simulink model "Disturbance_Stabilization_Simulink_Offline_Pendulum_Control"  (R2022b)
settings: Solver=VariableStepAuto  StartTime=0.0  StopTime=30  RelTol=1e-3
undefined symbols (not defined in the file): A, A_ob, B, B_ob, C_full, C_ob, D_full, D_ob, Kpp, sigbuilder_block, voltage_max, x0
settings Model: Creator=utente  LastModifiedBy=federicocorso
settings SolverCC: AlgebraicLoopSolver=TrustRegion
settings DebuggingCC: UnconnectedInputMsg=warning  UnconnectedOutputMsg=warning  UnconnectedLineMsg=warning  SFMachineParentedDataDiag=warning
settings ModelReferenceCC: EnableRefExpFcnMdlSchedulingChecks=on

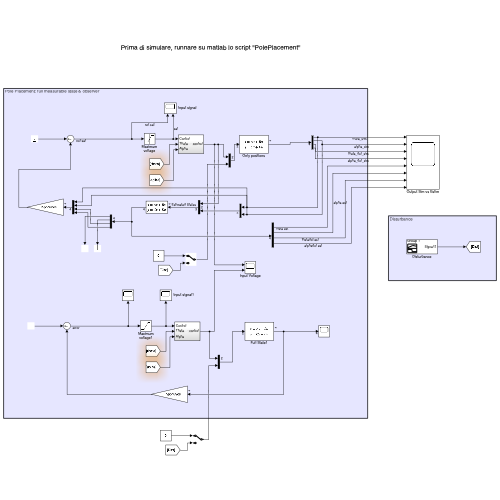
[thumbnail: Simulink's stored preview of the top-level diagram]
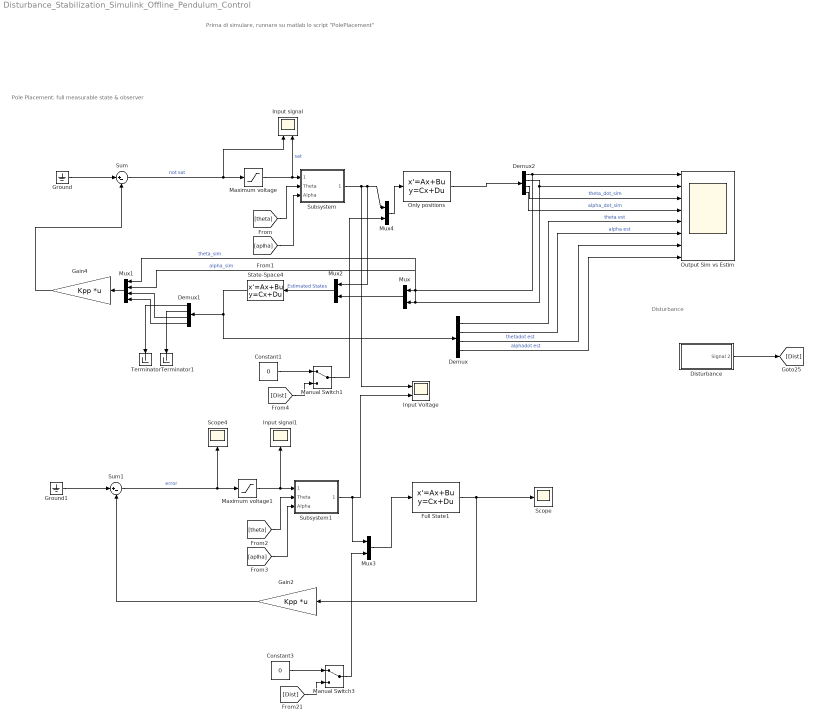
== system Disturbance_Stabilization_Simulink_Offline_Pendulum_Control ==
  note: Disturbance
  note: Pole Placement: full measurable state & observer
  note: Prima di simulare, runnare su matlab lo script "PolePlacement"
  Constant1 : Constant  Value=0
  Constant3 : Constant  Value=0
  Demux : Demux
  Demux1 : Demux
  Demux2 : Demux
  Disturbance : Subsystem  Tag=STV Subsys  LoadFcn=sigbuilder_block('load');  StartFcn=sigbuilder_block('start');  StopFcn=sigbuilder_block('stop');  ClipboardFcn=sigbuilder_block('clipboard');  mask(Sigbuilder block){tuvar=[0:10]}
      mask help: Simulink:masks:SigbuilderBlock_MD
      mask init:
      | if ~strcmp(get_param(bdroot(gcbh),'SimulationStatus'),'stopped') tuvar = sigbuilder_block('maskInit'); end
      settings: CopyFcn=sigbuilder_block('copy');  DeleteFcn=sigbuilder_block('delete');  ModelCloseFcn=sigbuilder_block('modelClose');  PreSaveFcn=sigbuilder_block('preSave');  PauseFcn=sigbuilder_block('pause');  ContinueFcn=sigbuilder_block('continue');  NameChangeFcn=sigbuilder_block('namechange');  OpenFcn=sigbuilder_block('open',[516 294 550 400 ]);  CloseFcn=sigbuilder_block('close');
      mask Display: plot(0, 0, 100, 100,[2, 2, 32, 32, 2], [68, 8, 8, 68, 68],[32, 2], [38, 38], [32, 19, 2],[53, 60, 44], [32, 17, 17, 2],[16, 16, 31, 31]);txt = getActiveGroup(gcbh);text(2, 100, txt,'verticalAlignment', 'top');
  Full State1 : StateSpace  A=A  B=B  C=C_full  D=D_full  InitialCondition=x0
  Gain2 : Gain  Gain=Kpp  Multiplication=Matrix(K*u) (u vector)
  Gain4 : Gain  Gain=Kpp  Multiplication=Matrix(K*u) (u vector)
  Ground : Ground
  Ground1 : Ground
  Input Voltage : Scope  NumInputPorts=2
  Input signal : Scope  NumInputPorts=2
  Input signal1 : Scope
  Manual Switch1 : ManualSwitch
  Manual Switch3 : ManualSwitch
  Maximum voltage : Saturate  UpperLimit=voltage_max  LowerLimit=-voltage_max
  Maximum voltage1 : Saturate  UpperLimit=voltage_max  LowerLimit=-voltage_max
  Mux{,2..4} (4 alike) : Mux  Inputs=2
  Mux1 : Mux
  Only positions : StateSpace  A=A  B=B  C=C_full  D=D_full  InitialCondition=x0
  Output Sim vs Estim : Scope  NumInputPorts=8
  Scope : Scope
  Scope4 : Scope
  State-Space4 : StateSpace  A=A_ob  B=B_ob  C=C_ob  D=D_ob  InitialCondition=[0;0;0;0]
  Subsystem : Subsystem
  Subsystem1 : Subsystem
  Sum : Sum  Inputs=|+-
  Sum1 : Sum  Inputs=|+-
  Terminator : Terminator
  Terminator1 : Terminator
  wires:
  Maximum voltage/1 -> Input signal/2, Subsystem/1(Control)  "sat"
  [theta] -> Subsystem/2(Theta)
  [aplha] -> Subsystem/3(Alpha)
  Ground/1 -> Sum/1
  Sum/1 -> Input signal/1, Maximum voltage/1  "not sat"
  Gain4/1 -> Sum/2
  Mux2/1 -> State-Space4/1  "Estimated States"
  State-Space4/1 -> Demux1/1, Demux/1
  Subsystem/1(control) -> Mux2/1, Mux4/1, Input Voltage/1
  Sum1/1 -> Maximum voltage1/1, Scope4/1  "error"
  Ground1/1 -> Sum1/1
  Full State1/1 -> Scope/1, Gain2/1
  Subsystem1/1(control) -> Input Voltage/2, Mux3/1
  Maximum voltage1/1 -> Input signal1/1, Subsystem1/1(Control)
  [aplha] -> Subsystem1/3(Alpha)
  [theta] -> Subsystem1/2(Theta)
  Gain2/1 -> Sum1/2
  Demux/1 -> Output Sim vs Estim/5  "theta est"
  Demux/2 -> Output Sim vs Estim/6  "alpha est"
  Demux/3 -> Output Sim vs Estim/7  "thetadot est"
  Demux/4 -> Output Sim vs Estim/8  "alphadot est"
  Only positions/1 -> Demux2/1
  Mux/1 -> Mux2/2
  Demux2/2 -> Output Sim vs Estim/2, Mux1/2, Mux/2  "alpha_sim"
  Demux2/1 -> Output Sim vs Estim/1, Mux1/1, Mux/1  "theta_sim"
  Demux2/3 -> Output Sim vs Estim/3  "theta_dot_sim"
  Demux2/4 -> Output Sim vs Estim/4  "alpha_dot_sim"
  Mux1/1 -> Gain4/1
  Demux1/3 -> Mux1/3
  Demux1/4 -> Mux1/4
  Demux1/1 -> Terminator/1
  Demux1/2 -> Terminator1/1
  Disturbance/1(Signal 2) -> [Dist]
  [Dist] -> Manual Switch3/2
  Manual Switch3/1 -> Mux3/2
  Constant3/1 -> Manual Switch3/1
  Mux3/1 -> Full State1/1
  Constant1/1 -> Manual Switch1/1
  [Dist] -> Manual Switch1/2
  Mux4/1 -> Only positions/1
  Manual Switch1/1 -> Mux4/2

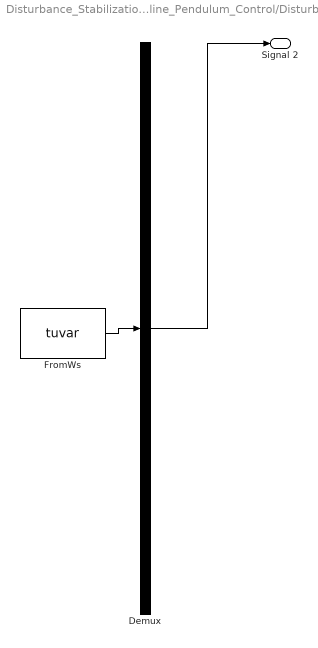
== system Disturbance_Stabilization_Simulink_Offline_Pendulum_Control/Disturbance ==
  Demux : Demux  Tag=STV Demux  Outputs=1
      settings: DisplayOption=none
  FromWs : FromWorkspace  Tag=STV FromWs  VariableName=tuvar
      SigBuilderData=|
      | common.afterFinalStr = 'Extrapolate'
      | common.sampleTime = 0
      | dataSet.timeRange = [0 10]
      | dataSet.name = 'Group 1'
      | sbobj.Groups.Name = 'Group 1'
      | sbobj.Groups.Signals.Name = 'Signal 2'
      | sbobj.Groups.Signals.XData = [0 4 4 4.01 4.01 10]
      | sbobj.Groups.Signals.YData = [0 0 0.2 0.2 0 0]
  Signal 2 : Outport  Tag=STV Outport
  wires:
  Demux/1 -> Signal 2/1
  FromWs/1 -> Demux/1

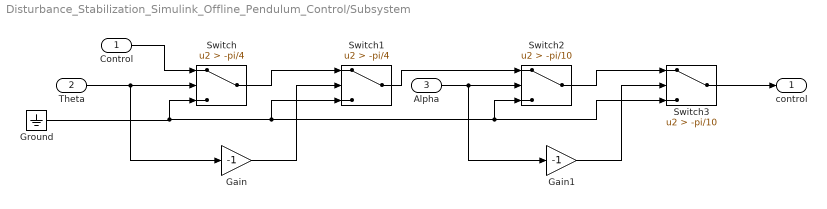
== system Disturbance_Stabilization_Simulink_Offline_Pendulum_Control/Subsystem ==
  Control : Inport
  Theta : Inport  Port=2
  Alpha : Inport  Port=3
  Gain : Gain  Gain=-1
  Gain1 : Gain  Gain=-1
  Ground : Ground
  Switch : Switch  Criteria=u2 > Threshold  Threshold=-pi/4  SaturateOnIntegerOverflow=off  InputSameDT=off
  Switch1 : Switch  Criteria=u2 > Threshold  Threshold=-pi/4  SaturateOnIntegerOverflow=off  InputSameDT=off
  Switch2 : Switch  Criteria=u2 > Threshold  Threshold=-pi/10  SaturateOnIntegerOverflow=off  InputSameDT=off
  Switch3 : Switch  Criteria=u2 > Threshold  Threshold=-pi/10  SaturateOnIntegerOverflow=off  InputSameDT=off
  control : Outport
  wires:
  Gain/1 -> Switch1/2
  Theta/1 -> Gain/1, Switch/2
  Control/1 -> Switch/1
  Switch/1 -> Switch1/1
  Gain1/1 -> Switch3/2
  Switch1/1 -> Switch2/1
  Ground/1 -> Switch3/3, Switch2/3, Switch1/3, Switch/3
  Switch2/1 -> Switch3/1
  Alpha/1 -> Switch2/2, Gain1/1
  Switch3/1 -> control/1

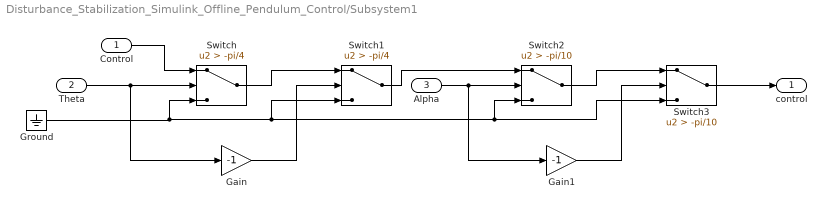
== system Disturbance_Stabilization_Simulink_Offline_Pendulum_Control/Subsystem1 ==
  Control : Inport
  Theta : Inport  Port=2
  Alpha : Inport  Port=3
  Gain : Gain  Gain=-1
  Gain1 : Gain  Gain=-1
  Ground : Ground
  Switch : Switch  Criteria=u2 > Threshold  Threshold=-pi/4  SaturateOnIntegerOverflow=off  InputSameDT=off
  Switch1 : Switch  Criteria=u2 > Threshold  Threshold=-pi/4  SaturateOnIntegerOverflow=off  InputSameDT=off
  Switch2 : Switch  Criteria=u2 > Threshold  Threshold=-pi/10  SaturateOnIntegerOverflow=off  InputSameDT=off
  Switch3 : Switch  Criteria=u2 > Threshold  Threshold=-pi/10  SaturateOnIntegerOverflow=off  InputSameDT=off
  control : Outport
  wires:
  Gain/1 -> Switch1/2
  Theta/1 -> Gain/1, Switch/2
  Control/1 -> Switch/1
  Switch/1 -> Switch1/1
  Gain1/1 -> Switch3/2
  Switch1/1 -> Switch2/1
  Ground/1 -> Switch3/3, Switch2/3, Switch1/3, Switch/3
  Switch2/1 -> Switch3/1
  Alpha/1 -> Switch2/2, Gain1/1
  Switch3/1 -> control/1
